simulink model "subsystem"  (R2024b)
settings: Solver=VariableStepAuto  StartTime=0.0  StopTime=10.0  RelTol=1e-3
libraries: simulink x3
settings Model: Creator=balaj  LastModifiedBy=balaj

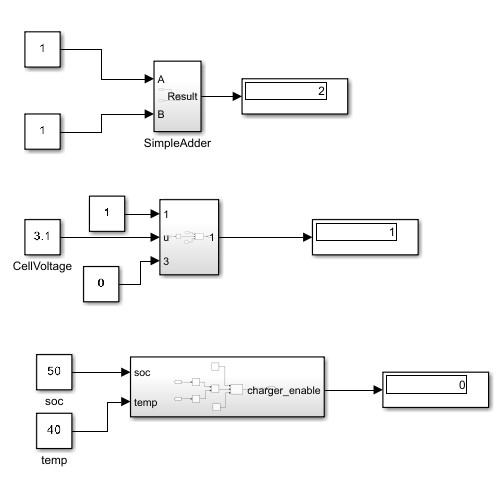
[thumbnail: Simulink's stored preview of the top-level diagram]
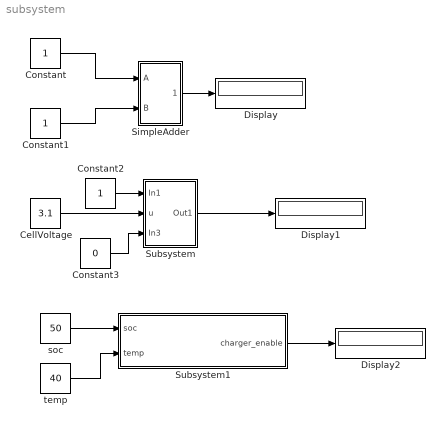
== system subsystem ==
  CellVoltage : Constant  Value=3.1
  Constant : Constant
  Constant1 : Constant
  Constant2 : Constant
  Constant3 : Constant  Value=0
  Display : Display
  Display1 : Display
  Display2 : Display
  SimpleAdder : Subsystem
  Subsystem : Subsystem
  Subsystem1 : Subsystem
  soc : Constant  Value=50
  temp : Constant  Value=40
  wires:
  Constant/1 -> SimpleAdder/1(A)
  Constant1/1 -> SimpleAdder/2(B)
  SimpleAdder/1(Result) -> Display/1
  Constant2/1 -> Subsystem/1(In1)
  CellVoltage/1 -> Subsystem/2(u)
  Constant3/1 -> Subsystem/3(In3)
  Subsystem/1(Out1) -> Display1/1
  soc/1 -> Subsystem1/1(soc)
  temp/1 -> Subsystem1/2(temp)
  Subsystem1/1(charger_enable) -> Display2/1

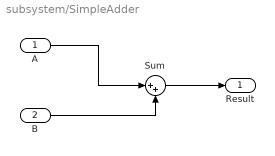
== system subsystem/SimpleAdder ==
  A : Inport
  B : Inport  Port=2
  Sum : Sum  Inputs=|++
  Result : Outport
  wires:
  Sum/1 -> Result/1
  A/1 -> Sum/1
  B/1 -> Sum/2

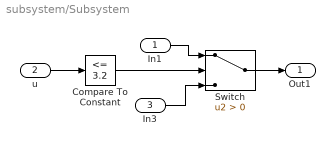
== system subsystem/Subsystem ==
  In1 : Inport
  u : Inport  Port=2
  In3 : Inport  Port=3
  Compare To Constant : simulink/Logic and Bit Operations/Compare To Constant  relop=<=  const=3.2  OutDataTypeStr=boolean
  Switch : Switch  Criteria=u2 > Threshold  SaturateOnIntegerOverflow=off  InputSameDT=off
  Out1 : Outport
  wires:
  In3/1 -> Switch/3
  Compare To Constant/1 -> Switch/2
  Switch/1 -> Out1/1
  In1/1 -> Switch/1
  u/1 -> Compare To Constant/1

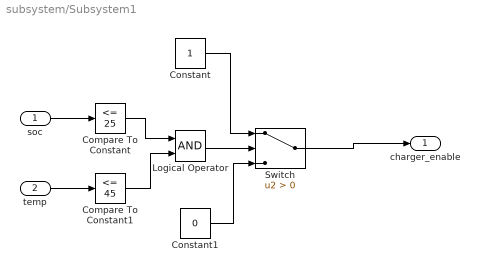
== system subsystem/Subsystem1 ==
  soc : Inport
  temp : Inport  Port=2
  Compare To Constant : simulink/Logic and Bit Operations/Compare To Constant  relop=<=  const=25  OutDataTypeStr=boolean
  Compare To Constant1 : simulink/Logic and Bit Operations/Compare To Constant  relop=<=  const=45  OutDataTypeStr=boolean
  Constant : Constant
  Constant1 : Constant  Value=0
  Logical Operator : Logic  AllPortsSameDT=off  OutDataTypeStr=boolean
  Switch : Switch  Criteria=u2 > Threshold  SaturateOnIntegerOverflow=off  InputSameDT=off
  charger_enable : Outport
  wires:
  soc/1 -> Compare To Constant/1
  temp/1 -> Compare To Constant1/1
  Compare To Constant/1 -> Logical Operator/1
  Compare To Constant1/1 -> Logical Operator/2
  Logical Operator/1 -> Switch/2
  Constant/1 -> Switch/1
  Constant1/1 -> Switch/3
  Switch/1 -> charger_enable/1
